simulink model "power_KundurTwoAreaSystem__RTLAB"  (R2021b)
settings: Solver=ode4  StartTime=0.0  StopTime=15  FixedStep=Ts  MaxStep=1/60  RelTol=1e-4
PostLoadFcn:
  | Ts=50e-6; PSSMODEL=1
InitFcn:
  | Ts=50e-6; PSSMODEL=1
undefined symbols (not defined in the file): D1, Delta
libraries: spsGenericPowerSystemStabilizerLib x8, spsThreePhaseVIMeasurementLib x6, spsLoadFlowBusLib x6, spsThreePhaseParallelRLCLoadLib x4, spsThreePhasePISectionLineLib x4, spsSynchronousMachinepuStandardLib x4, spsExcitationSystemLib x4, spsSteamTurbineandGovernorLib x4, spsThreePhaseSeriesRLCLoadLib x4, spsThreePhaseTransformerTwoWindingsLib x4, spsThreePhaseBreakerLib x2, op_dpl_lib x2
(part 1 of 2)
settings Model: ARTEMISmethode_block_infos=$$__separator__$$power_KundurTwoAreaSystem/ARTEMIS Guide$$__separator__$$  Creator=The MathWorks, Inc.  LastModifiedBy=Real_LAB
settings SolverCC: AlgebraicLoopSolver=TrustRegion
settings DataIOCC: SaveOutput=off  SignalLogging=off  DSMLogging=off  SaveTime=off  ReturnWorkspaceOutputs=off  TimeSaveName=t  SignalLoggingName=sigsOut
settings OptimizationCC: BlockReduction=off  BooleanDataType=off  OptimizeBlockIOStorage=off  BufferReuse=off  GlobalBufferReuse=off  ExpressionFolding=off  ExpressionDepthLimit=2147483647  LocalBlockOutputs=off  InitFltsAndDblsToZero=on  LifeSpan=inf  OptimizeDataStoreBuffers=off  BusAssignmentInplaceUpdate=off
settings DebuggingCC: SaveWithParameterizedLinksMsg=none  SignalResolutionControl=TryResolveAllWithWarning  MultiTaskDSMMsg=warning  MultiTaskCondExecSysMsg=none  FcnCallInpInsideContextMsg=warning  UnconnectedOutputMsg=none  StateNameClashWarn=warning  SFUnexpectedBacktrackingDiag=warning  SFNoUnconditionalDefaultTransitionDiag=warning  SFExecutionAtInitializationDiag=none  SFMachineParentedDataDiag=warning  ArithmeticOperatorsInVariantConditions=warning
settings HardwareCC: ProdBitPerPointer=32  ProdBitPerSizeT=32  ProdBitPerPtrDiffT=32  ProdLargestAtomicFloat=None  ProdIntDivRoundTo=Undefined  ProdEndianess=Unspecified  ProdWordSize=32  ProdHWDeviceType=32-bit Generic  TargetBitPerPointer=64  TargetBitPerSizeT=64  TargetBitPerPtrDiffT=64  TargetLongLongMode=on  TargetIntDivRoundTo=Zero  TargetEndianess=LittleEndian  TargetWordSize=64  TargetHWDeviceType=MATLAB Host  ProdEqTarget=off
settings ModelReferenceCC: PropagateSignalLabelsOutOfModel=off
settings SFSimCC: SimUseLocalCustomCode=off  CustomCodeUndefinedFunction=UseInterfaceOnly
settings RTWCC: RTWUseLocalCustomCode=off
settings CodeAppCC: StateflowObjectComments=on
settings GRTTargetCC: TargetFcnLib=ansi_tfl_tmw.mat  TargetLangStandard=C89/C90 (ANSI)  CombineOutputUpdateFcns=off  GRTInterface=on
settings ConfigComp: CovMetricSettings=dw  CovSaveCumulativeToWorkspaceVar=on  CovSaveSingleToWorkspaceVar=on  CovExternalEMLEnable=off  CovSFcnEnable=off
settings SimscapeCC: SimscapeNormalizeSystem=off  SimscapeNominalValues={1, 'bar'; 1, 'cm^3/s'; 1, 'bar*kg/s'; 1, 'kJ/kg'; 1, 'kW'; }

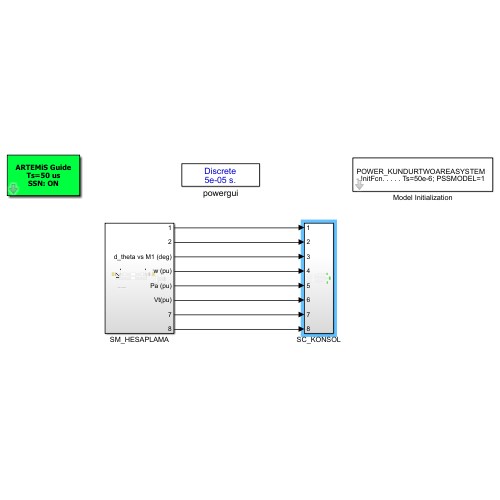
[thumbnail: Simulink's stored preview of the top-level diagram]
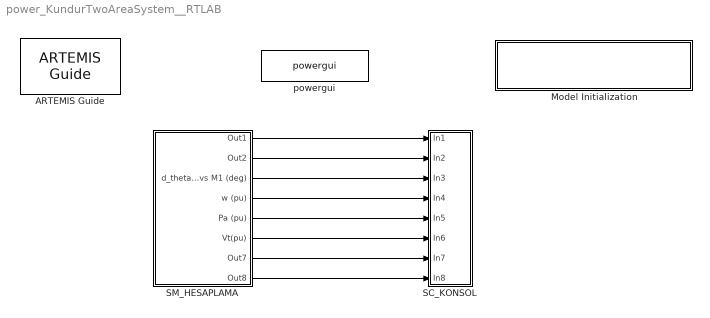
== system power_KundurTwoAreaSystem__RTLAB ==
  ARTEMIS Guide : artemis/ARTEMIS/ARTEMIS Guide  Tag=art7.5  Description=New ARTEMiS block v 7.5b (R2015b+)  lock=on  Ts=Ts  ssn=on  opt=art5  dyna=off  nb_perm=4  RT_fullcomp=off  ssn_itvc=off  ssn_ivic=off  ssn_ext=off  ssn_solver=Art5  iter_type=iSWITCH and iMOV only (default)  ssn_ImpulseLoopBlockedStateUpdate=5  ssn_mov_iter_number=5  ssn_switch_iter_number=3  ssn_lu_or_ldlt=LU (more robust)  ssn_nib_type_verify=on  ssn_use_lu=on  ssn_use_ldlt=off  ssn_impulse=on  ssn_quasimpulse=off  ssn_impulse_loop=5  paraExtinctionThy=off  Thy_Impulse=on  dtc=Off  dtc_opt=normal  ao=off  simtype=off  ct_mac=off  lin_mov=off  lsp=[0.001 2]  spike_skip=Disabled  dtc_extra=1  dtc_sws=normal  dtc_pied=0.5  SPSRulesBlock=SPSRules  tre=off  ctmm=off  LF=off  dpl_type=ARTEMiS DPL  rlc_type=off  custom_type=off  para=on  ssn_full_iteration=off  ssn_init_cond=block only
  Model Initialization : Subsystem  AncestorBlock=artemis/Tools /Misc/Model Initialization  mask(Model Functions){InitFcnX=Ts=50e-6; PSSMODEL=1, prel=off, posl=on, inif=on, strf=off}
      mask prompts: InitFcnX "Initialisation"; prel "Preload Function"; posl "PostLoad Function"; inif "InitFcn"; strf "StartFcn"
      mask init:
      | currentBlock = gcb;
      | root = bdroot(currentBlock);
      | 
      | if ~strcmp(get_param(root,'BlockDiagramType'),'library')
      |     if prel==1
      |         set_param(root, 'PreLoadFcn', InitFcnX);
      |     else
      |         set_param(root, 'PreLoadFcn', '');
      |     end
      |     if inif==1
      |         set_param(root, 'InitFcn', InitFcnX);
      |     else
      |         set_param(root, 'InitFcn', '');
      |     end
      |     if strf==1
      |         set_param(root, 'StartFcn', InitFcnX);
      |     else
      |         set_param(root, 'StartFcn', '');
      |     end
      |     if posl==1
      |         set_param(root, 'PostLoadFcn', InitFcnX);
      |     else
      |         set_param(root, 'PostLoadFcn', '');
      |     end
      | end
      | 
      | pos = get_param(currentBlock, 'Position');
      | width = pos(3) - pos(1); height = pos(4) - pos(2);
      | txt = [ upper(root) '\n' '- InitFcn. . . . . '  get_param(root, 'InitFcn') ];
      settings: CopyFcn=set_param(gcb,'LinkStatus','inactive')
      mask Display: text(5, height*0.5, txt, 'horizontalAlignment', 'left', 'verticalAlignment', 'middle') ;
  SC_KONSOL : Subsystem
  SM_HESAPLAMA : Subsystem
  powergui : spspowerguiLib/powergui  Priority=2  SimulationMode=Discrete  SampleTime=Ts  frequency=60  Iterations=50  frequencyindice=60  Pbase=100e6  ErrMax=1e-4  UnitsV=kV  UnitsW=MW  buscounter=0  FunctionMessages=off  echomessages=off  EnableUseOfTLC=off  CurrentSourceSwitches=off  DisableSnubberDevices=off  DisableRonSwitches=off  DisableVfSwitches=off  DisplayEquations=off  AutomaticDiscreteSolvers=off  SolverType=Tustin  Interpol=off  ExternalGateDelay=off  methode=off  Ts=0  x0status=blocks  SPID=off  SwTol=0  HookPort=off  NonlinearTolerance=1e-4  nMaxIteration=100  ContinueOnMaxIteration=off  RestoreLinks=warning  ResistiveCurrentMeasurement=off  Frange=logspace(0,3,50)  Ylog=off  Xlog=off  ShowGrid=off  save=off  variable=ZData  structure=0  ZoomFFT=on  StartTime=0.0  cycles=1  DisplayStyle=1  fundamental=60  FreqAxis=off  MaxFrequency=1000  frequencyindicesteady=1  RmsSteady=1  display=off
  wires:
  SM_HESAPLAMA/1(Out1) -> SC_KONSOL/1(In1)
  SM_HESAPLAMA/2(Out2) -> SC_KONSOL/2(In2)
  SM_HESAPLAMA/3(d_theta vs M1 (deg)) -> SC_KONSOL/3(In3)
  SM_HESAPLAMA/4(w (pu)) -> SC_KONSOL/4(In4)
  SM_HESAPLAMA/5(Pa (pu)) -> SC_KONSOL/5(In5)
  SM_HESAPLAMA/6(Vt(pu)) -> SC_KONSOL/6(In6)
  SM_HESAPLAMA/7(Out7) -> SC_KONSOL/7(In7)
  SM_HESAPLAMA/8(Out8) -> SC_KONSOL/8(In8)

== system power_KundurTwoAreaSystem__RTLAB/Model Initialization ==

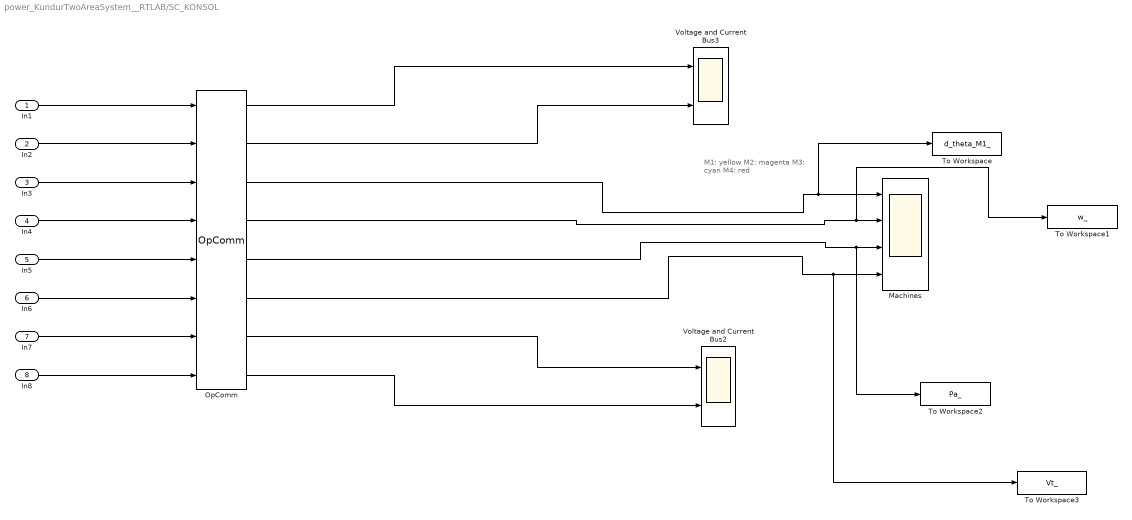
== system power_KundurTwoAreaSystem__RTLAB/SC_KONSOL ==
  note: M1: yellow
      | M2: magenta
      | M3: cyan
      | M4: red
  In1 : Inport
  In2 : Inport  Port=2
  In3 : Inport  Port=3
  In4 : Inport  Port=4
  In5 : Inport  Port=5
  In6 : Inport  Port=6
  In7 : Inport  Port=7
  In8 : Inport  Port=8
  Machines : Scope  NumInputPorts=4
  OpComm : rtlab/OpComm  nbport=8  groupe_acq=1  subsys_rate=0  st=0  Synchronization=on  Interpolation=on  Threshold=1.0  Missed_Data=off  Sim_Time=off  Samples=off  dynSigOut=off  from_console=0  warning_done=off  writeOpCommFile=off  Offset=off
      settings: SourceProductName=RT-LAB
  To Workspace : ToWorkspace  VariableName=d_theta_M1_  SaveFormat=Timeseries  SampleTime=-1
  To Workspace1 : ToWorkspace  VariableName=w_  SaveFormat=Timeseries  SampleTime=-1
  To Workspace2 : ToWorkspace  VariableName=Pa_  SaveFormat=Timeseries  SampleTime=-1
  To Workspace3 : ToWorkspace  VariableName=Vt_  SaveFormat=Timeseries  SampleTime=-1
  Voltage and Current Bus2 : Scope  NumInputPorts=2
  Voltage and Current Bus3 : Scope  NumInputPorts=2
  wires:
  In1/1 -> OpComm/1
  In2/1 -> OpComm/2
  In3/1 -> OpComm/3
  In4/1 -> OpComm/4
  In5/1 -> OpComm/5
  In6/1 -> OpComm/6
  In7/1 -> OpComm/7
  In8/1 -> OpComm/8
  OpComm/8 -> Voltage and Current Bus2/2
  OpComm/7 -> Voltage and Current Bus2/1
  OpComm/1 -> Voltage and Current Bus3/1
  OpComm/2 -> Voltage and Current Bus3/2
  OpComm/3 -> To Workspace/1, Machines/1
  OpComm/4 -> To Workspace1/1, Machines/2
  OpComm/5 -> To Workspace2/1, Machines/3
  OpComm/6 -> To Workspace3/1, Machines/4

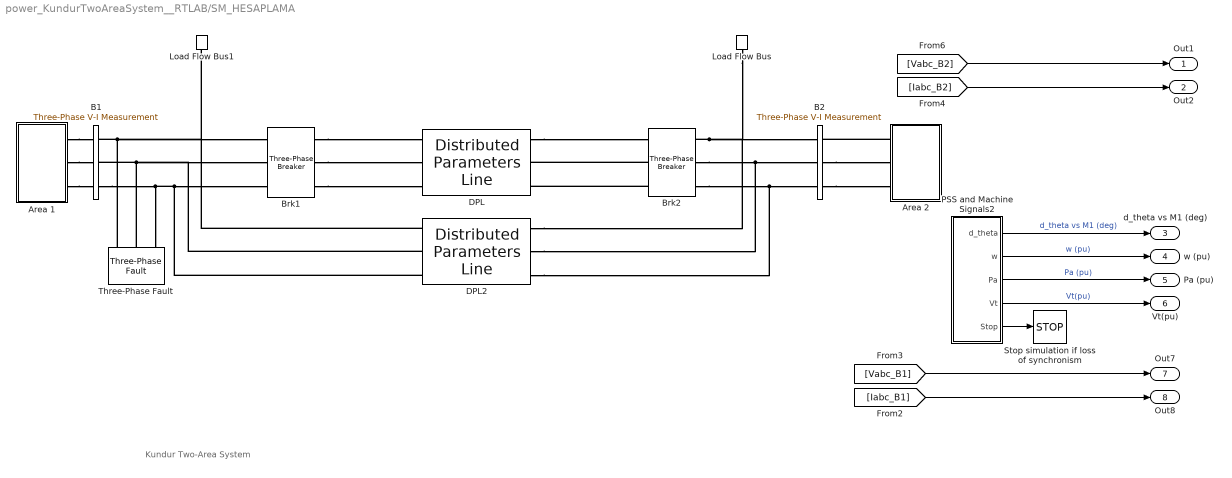
== system power_KundurTwoAreaSystem__RTLAB/SM_HESAPLAMA ==
  note: Kundur Two-Area System
  " Brk2" : spsThreePhaseBreakerLib/Three-Phase Breaker  InitialState=closed  SwitchA=on  SwitchB=on  SwitchC=on  SwitchTimes=[2+12]*100  External=off  BreakerResistance=0.001  SnubberResistance=1e6  SnubberCapacitance=0  Measurements=None
      settings: AttributesFormatString=\n
  Area 1 : Subsystem
  Area 2 : Subsystem
  B1 : spsThreePhaseVIMeasurementLib/Three-Phase V-I Measurement  VoltageMeasurement=phase-to-ground  SetLabelV=on  LabelV=Vabc_B1  Vpu=on  VpuLL=off  CurrentMeasurement=yes  SetLabelI=on  LabelI=Iabc_B1  Ipu=off  Pbase=100e6  Vbase=230e3  OutputType=Complex  PhasorSimulation=off  PSBequivalent=0
  B2 : spsThreePhaseVIMeasurementLib/Three-Phase V-I Measurement  VoltageMeasurement=phase-to-ground  SetLabelV=on  LabelV=Vabc_B2  Vpu=off  VpuLL=off  CurrentMeasurement=yes  SetLabelI=on  LabelI=Iabc_B2  Ipu=off  Pbase=100e6  Vbase=500e3  OutputType=Complex  PhasorSimulation=off  PSBequivalent=0
  Brk1 : spsThreePhaseBreakerLib/Three-Phase Breaker  InitialState=closed  SwitchA=off  SwitchB=off  SwitchC=off  SwitchTimes=[2+12]  External=off  BreakerResistance=0.001  SnubberResistance=inf  SnubberCapacitance=0  Measurements=None
      settings: AttributesFormatString=\n
  DPL : op_dpl_lib/Distributed Parameters Line  SimulationMode=ARTEMIS model  Phases=3  Frequency=60  Resistance=[0.0001*529 1.61]  Inductance=[0.001*529/(377) 0.0061]  Capacitance=[0.00175/529/(377) 5.2489e-9]  Length=220  Measurements=None
  DPL2 : op_dpl_lib/Distributed Parameters Line  SimulationMode=ARTEMIS model  Phases=3  Frequency=60  Resistance=[0.0001*529 1.61]  Inductance=[0.001*529/(377) 0.0061]  Capacitance=[0.00175/529/(377) 5.2489e-9]  Length=220  Measurements=None
  Load Flow Bus : spsLoadFlowBusLib/Load Flow Bus  LConnTagsString=a  Phases=single  Connectors=on one side  ID=B2  Vbase=230e3  Vref=1  Vangle=0  VLF=1.003  VLFb=1  VLFc=1  angleLF=-11.54  angleLFb=0  angleLFc=0
      settings: AttributesFormatString=%<ID>\n%<Vbase>V\n%<VLF>pu\n%<angleLF>deg.  SourceProductBaseCode=PS
  Load Flow Bus1 : spsLoadFlowBusLib/Load Flow Bus  LConnTagsString=a  Phases=single  Connectors=on one side  ID=B1  Vbase=230e3  Vref=1  Vangle=0  VLF=0.9914  VLFb=1  VLFc=1  angleLF=15.04  angleLFb=0  angleLFc=0
      settings: AttributesFormatString=%<ID>\n%<Vbase>V\n%<VLF>pu\n%<angleLF>deg.  SourceProductBaseCode=PS
  PSS and Machine Signals2 : Subsystem
  Stop simulation if loss of synchronism : Stop
  Three-Phase Fault : spsThreePhaseFaultLib/Three-Phase Fault  InitialStates=0  FaultA=on  FaultB=on  FaultC=on  GroundFault=on  SwitchTimes=[2 2.1]  External=off  SwitchStatus=NaN  FaultResistance=0.001  GroundResistance=0.001  SnubberResistance=1e6  SnubberCapacitance=inf  Measurements=None
  Out1 : Outport
  Out2 : Outport  Port=2
  d_theta vs M1 (deg) : Outport  Port=3
  w (pu) : Outport  Port=4
  Pa (pu) : Outport  Port=5
  Vt(pu) : Outport  Port=6
  Out7 : Outport  Port=7
  Out8 : Outport  Port=8
  wires:
  [Vabc_B2] -> Out1/1
  PSS and Machine Signals2/1(d_theta) -> d_theta vs M1 (deg)/1  "d_theta vs M1 (deg)"
  PSS and Machine Signals2/4(Vt) -> Vt(pu)/1  "Vt(pu)"
  PSS and Machine Signals2/2(w) -> w (pu)/1  "w (pu)"
  PSS and Machine Signals2/5(Stop) -> Stop simulation if loss of synchronism/1
  [Iabc_B1] -> Out8/1
  [Vabc_B1] -> Out7/1
  [Iabc_B2] -> Out2/1
  PSS and Machine Signals2/3(Pa) -> Pa (pu)/1  "Pa (pu)"
  connections:
  B2/RConn2 -- Area 2/LConn2
  " Brk2"/LConn2 -- DPL/RConn2
  B2/RConn3 -- Area 2/LConn3
  " Brk2"/RConn1 -- DPL2/RConn1 -- Load Flow Bus/LConn1 -- B2/LConn1
  " Brk2"/RConn2 -- DPL2/RConn2 -- B2/LConn2
  Area 1/RConn3 -- B1/LConn3
  Area 1/RConn1 -- B1/LConn1
  Brk1/RConn3 -- DPL/LConn3
  DPL2/LConn1 -- Brk1/LConn1 -- Load Flow Bus1/LConn1 -- Three-Phase Fault/LConn1 -- B1/RConn1
  Brk1/RConn1 -- DPL/LConn1
  Area 2/LConn1 -- B2/RConn1
  DPL2/LConn3 -- B1/RConn3 -- Three-Phase Fault/LConn3 -- Brk1/LConn3
  " Brk2"/LConn3 -- DPL/RConn3
  " Brk2"/RConn3 -- DPL2/RConn3 -- B2/LConn3
  DPL/RConn1 -- " Brk2"/LConn1
  DPL2/LConn2 -- Brk1/LConn2 -- Three-Phase Fault/LConn2 -- B1/RConn2
  Brk1/RConn2 -- DPL/LConn2
  Area 1/RConn2 -- B1/LConn2

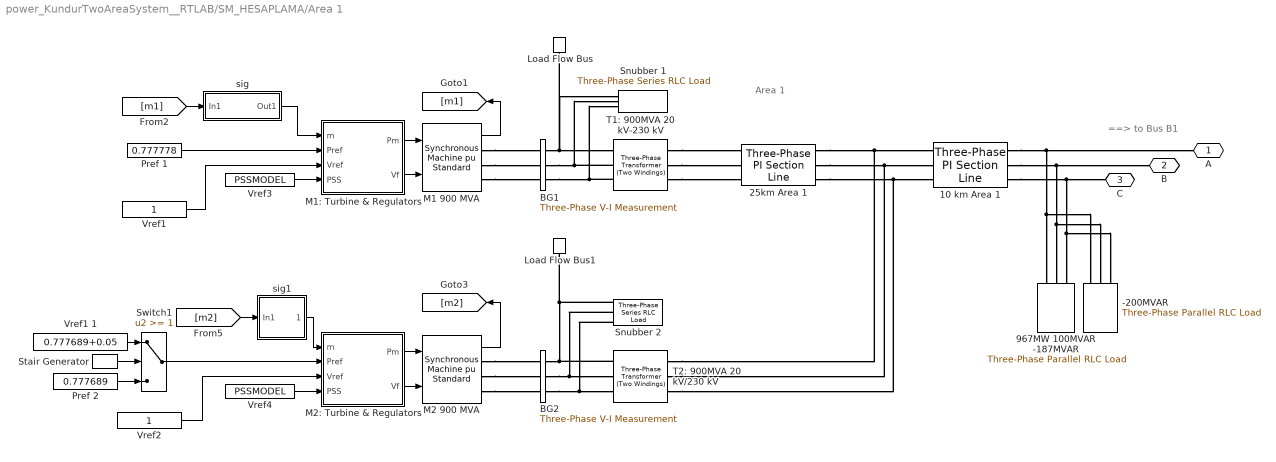
== system power_KundurTwoAreaSystem__RTLAB/SM_HESAPLAMA/Area 1 ==
  note: Area 1
  note: ==> to Bus B1
  -200MVAR : spsThreePhaseParallelRLCLoadLib/Three-Phase Parallel RLC Load  LConnTagsString=A|B|C  Configuration=Y (grounded)  NominalVoltage=230e3  Vabc=[1e3 1e3 1e3]  Vabcp=[1e3 1e3 1e3]  NominalFrequency=60  UnbalancedPower=off  ActivePower=0  InductivePower=0  CapacitivePower=200e6  Pabc=[10e3 9e3 11e3]  QLabc=[100 90 110]  QCabc=[100 90 110]  Pabcp=[10e3 9e3 11e3]  QLabcp=[100 90 110]  QCabcp=[100 90 110]  Measurements=None  LoadType=constant Z
  10 km Area 1 : spsThreePhasePISectionLineLib/Three-Phase PI Section Line  LConnTagsString=a|b|c  RConnTagsString=A|B|C  Length=10  Frequency=60  Resistances=[0.0001*529 1.61]  Inductances=[0.001*529/(377) 0.0061]  Capacitances=[0.00175/529/(377) 5.2489e-9]
  25km Area 1 : spsThreePhasePISectionLineLib/Three-Phase PI Section Line  LConnTagsString=a|b|c  RConnTagsString=A|B|C  Length=25  Frequency=60  Resistances=[0.0001*529 1.61]  Inductances=[0.001*529/(377) 0.0061]  Capacitances=[0.00175/529/(377) 5.2489e-9]
  967MW 100MVAR -187MVAR : spsThreePhaseParallelRLCLoadLib/Three-Phase Parallel RLC Load  LConnTagsString=A|B|C  Configuration=Y (grounded)  NominalVoltage=230e3  Vabc=[1e3 1e3 1e3]  Vabcp=[1e3 1e3 1e3]  NominalFrequency=60  UnbalancedPower=off  ActivePower=967e6  InductivePower=100e6  CapacitivePower=187e6  Pabc=[10e3 9e3 11e3]  QLabc=[100 90 110]  QCabc=[100 90 110]  Pabcp=[10e3 9e3 11e3]  QLabcp=[100 90 110]  QCabcp=[100 90 110]  Measurements=None  LoadType=constant Z
  BG1 : spsThreePhaseVIMeasurementLib/Three-Phase V-I Measurement  VoltageMeasurement=phase-to-ground  SetLabelV=on  LabelV=Vabc_G1  Vpu=on  VpuLL=off  CurrentMeasurement=yes  SetLabelI=on  LabelI=Iabc_G1  Ipu=on  Pbase=900e6  Vbase=20e3  OutputType=Complex  PhasorSimulation=off  PSBequivalent=0
  BG2 : spsThreePhaseVIMeasurementLib/Three-Phase V-I Measurement  VoltageMeasurement=no  SetLabelV=on  LabelV=Vabc_G2  Vpu=on  VpuLL=off  CurrentMeasurement=no  SetLabelI=on  LabelI=Iabc_G2  Ipu=on  Pbase=900e6  Vbase=20e3  OutputType=Complex  PhasorSimulation=off  PSBequivalent=0
  Load Flow Bus : spsLoadFlowBusLib/Load Flow Bus  LConnTagsString=a  Phases=single  Connectors=on one side  ID=M1_Area1  Vbase=20e3  Vref=1  Vangle=0  VLF=1  VLFb=1  VLFc=1  angleLF=10.19  angleLFb=0  angleLFc=0
      settings: AttributesFormatString=%<ID>\n%<Vbase>V\n%<VLF>pu\n%<angleLF>deg.  SourceProductBaseCode=PS
  Load Flow Bus1 : spsLoadFlowBusLib/Load Flow Bus  LConnTagsString=a  Phases=single  Connectors=on one side  ID=M2_Area1  Vbase=20e3  Vref=1  Vangle=0  VLF=1  VLFb=1  VLFc=1  angleLF=0  angleLFb=0  angleLFc=0
      settings: AttributesFormatString=%<ID>\n%<Vbase>V\n%<VLF>pu\n%<angleLF>deg.  SourceProductBaseCode=PS
  M1 900 MVA : spsSynchronousMachinepuStandardLib/Synchronous Machine pu Standard  PresetModel=No  MechanicalLoad=Mechanical power Pm  ShowDetailedParameters=on  RotorType=Round  Units=per unit standard parameters  MeasurementBus=off  NominalParameters="[900E6  20000   60 ]"  Reactances1=[1.8 .3 .25 1.7 .55 .25 .2]  Reactances2=[ 1.305, 0.296, 0.252, 0.474, 0.243, 0.18 ]  dAxisTimeConstants=Open-circuit  qAxisTimeConstants=Open-circuit  TimeConstants1=[]  TimeConstants2=[8 .03 .4 .05]  TimeConstants3=[]  TimeConstants4=[]  TimeConstants5=[ 1.01, 0.053, 0.1 ]  TimeConstants6=[]  TimeConstants7=[]  TimeConstants8=[]  StatorResistance=0.0025  Mechanical="[ 6.5 0  4]"  PolePairs=4  InitialConditions=[0 -31.4247 0.784453 0.784453 0.784453 2.7401 -117.26 122.74 1.83395]  SetSaturation=off  Saturation=[0.6404,0.7127,0.8441,0.9214,0.9956,1.082,1.19,1.316,1.457;0.7,0.7698,0.8872,0.9466,0.9969,1.046,1.1,1.151,1.201]  LoadFlowParameters=[1 700000000 0 0 0]  TsPowergui=0  TsBlock=-1  IterativeModel=Trapezoidal non iterative  IterativeDiscreteModel=Trapezoidal non iterative  BusType=PV  Pref=700000000  Qref=0  Qmin=-inf  Qmax=inf  PLF=0  QLF=0
      settings: SourceProductBaseCode=PS
  M1: Turbine & Regulators : Subsystem
  M2 900 MVA : spsSynchronousMachinepuStandardLib/Synchronous Machine pu Standard  PresetModel=No  MechanicalLoad=Mechanical power Pm  ShowDetailedParameters=on  RotorType=Round  Units=per unit standard parameters  MeasurementBus=off  NominalParameters="[900E6  20000   60 ]"  Reactances1=[1.8 .3 .25 1.7 .55 .25 .2]  Reactances2=[ 1.305, 0.296, 0.252, 0.474, 0.243, 0.18 ]  dAxisTimeConstants=Open-circuit  qAxisTimeConstants=Open-circuit  TimeConstants1=[]  TimeConstants2=[8 .03 .4 .05]  TimeConstants3=[]  TimeConstants4=[]  TimeConstants5=[ 1.01, 0.053, 0.1 ]  TimeConstants6=[]  TimeConstants7=[]  TimeConstants8=[]  StatorResistance=0.0025  Mechanical="[ 6.5 0  4]"  PolePairs=4  InitialConditions=[0 -42.8075 0.788608 0.788608 0.788608 -9.54571 -129.546 110.454 1.86756]  SetSaturation=off  Saturation=[0.6404,0.7127,0.8441,0.9214,0.9956,1.082,1.19,1.316,1.457;0.7,0.7698,0.8872,0.9466,0.9969,1.046,1.1,1.151,1.201]  LoadFlowParameters=[2 700000000 0 0 0]  TsPowergui=0  TsBlock=-1  IterativeModel=Trapezoidal non iterative  IterativeDiscreteModel=Trapezoidal non iterative  BusType=swing  Pref=0  Qref=0  Qmin=-inf  Qmax=inf  PLF=0  QLF=0
      settings: SourceProductBaseCode=PS
  M2: Turbine & Regulators : Subsystem
  Pref 1 : Constant  Value=0.777778
  Pref 2 : Constant  Value=0.777689
  Snubber 1 : spsThreePhaseSeriesRLCLoadLib/Three-Phase Series RLC Load  LConnTagsString=A|B|C  Configuration=Y (grounded)  NominalVoltage=20000  Vabc=[1e3 1e3 1e3]  Vabcp=[1e3 1e3 1e3]  NominalFrequency=60  UnbalancedPower=off  ActivePower=1e6  InductivePower=0  CapacitivePower=1e7  Pabc=[10e3 9e3 11e3]  QLabc=[100 90 110]  QCabc=[100 90 110]  Pabcp=[10e3 9e3 11e3]  QLabcp=[100 90 110]  QCabcp=[100 90 110]  Measurements=None  LoadType=constant Z
  Snubber 2 : spsThreePhaseSeriesRLCLoadLib/Three-Phase Series RLC Load  LConnTagsString=A|B|C  Configuration=Y (grounded)  NominalVoltage=20000  Vabc=[1e3 1e3 1e3]  Vabcp=[1e3 1e3 1e3]  NominalFrequency=60  UnbalancedPower=off  ActivePower=1e6  InductivePower=0  CapacitivePower=1e7  Pabc=[10e3 9e3 11e3]  QLabc=[100 90 110]  QCabc=[100 90 110]  Pabcp=[10e3 9e3 11e3]  QLabcp=[100 90 110]  QCabcp=[100 90 110]  Measurements=None  LoadType=constant Z
  Stair Generator : spsStairGeneratorLib/Stair Generator  t=[0 15 20]  e=[0 1 0 ]  Ts=0
  Switch1 : Switch  Threshold=1  InputSameDT=on
  T1: 900MVA 20 kV-230 kV : spsThreePhaseTransformerTwoWindingsLib/Three-Phase Transformer (Two Windings)  Winding1Connection=Delta (D1)  Winding2Connection=Yg  CoreType=Three single-phase transformers  SetSaturation=off  Hysteresis=off  DataFile='hysteresis'  SetInitialFlux=off  Measurements=None  UNITS=pu  NominalPower="[ 900e6   60 ]"  Winding1="[ 20e3  1e-6   0  ]"  Winding2="[ 230e3  1e-6   0.15 ]"  Rm=500  Lm=500  L0=0.5  Saturation="[ 0,0  ;  0.005,1.2  ;  1.0,1.4 ]"  InitialFluxes=[ 0.8 , -0.8 , 0.7 ]  BreakLoop=off  DiscreteSolver=Trapezoidal iterative  DataType=off  TransfoNumber=0
  T2: 900MVA 20 kV/230 kV : spsThreePhaseTransformerTwoWindingsLib/Three-Phase Transformer (Two Windings)  Winding1Connection=Delta (D1)  Winding2Connection=Yg  CoreType=Three single-phase transformers  SetSaturation=off  Hysteresis=off  DataFile='hysteresis'  SetInitialFlux=off  Measurements=None  UNITS=pu  NominalPower=[ 900e6 60 ]  Winding1="[ 20e3 1e-6  0.0]"  Winding2=[ 230e3 1e-6 0.15]  Rm=500  Lm=500  L0=0.5  Saturation="[ 0,0  ;  0.005,1.2  ;  1.0,1.4 ]"  InitialFluxes=[ 0.8 , -0.8 , 0.7 ]  BreakLoop=off  DiscreteSolver=Trapezoidal iterative  DataType=off  TransfoNumber=0
  Vref1 : Constant
  Vref1 1 : Constant  Value=0.777689+0.05
  Vref2 : Constant
  Vref3 : Constant  Value=PSSMODEL
  Vref4 : Constant  Value=PSSMODEL
  sig : Subsystem
  sig1 : Subsystem
  " A" : PMIOPort  Side=Right
  " B" : PMIOPort  Port=2  Side=Right
  " C" : PMIOPort  Port=3  Side=Right
  wires:
  Pref 1/1 -> M1: Turbine & Regulators/2(Pref)
  Vref2/1 -> M2: Turbine & Regulators/3(Vref)
  Vref4/1 -> M2: Turbine & Regulators/4(PSS)
  sig/1(Out1) -> M1: Turbine & Regulators/1(m)
  M1 900 MVA/1 -> [m1]
  M2 900 MVA/1 -> [m2]
  [m1] -> sig/1(In1)
  Vref3/1 -> M1: Turbine & Regulators/4(PSS)
  sig1/1(Out1) -> M2: Turbine & Regulators/1(m)
  [m2] -> sig1/1(In1)
  Stair Generator/1 -> Switch1/2
  Pref 2/1 -> Switch1/3
  Vref1 1/1 -> Switch1/1
  Switch1/1 -> M2: Turbine & Regulators/2(Pref)
  Vref1/1 -> M1: Turbine & Regulators/3(Vref)
  M1: Turbine & Regulators/1(Pm) -> M1 900 MVA/1
  M1: Turbine & Regulators/2(Vf) -> M1 900 MVA/2
  M2: Turbine & Regulators/2(Vf) -> M2 900 MVA/2
  M2: Turbine & Regulators/1(Pm) -> M2 900 MVA/1
  connections:
  T1: 900MVA 20 kV-230 kV/RConn1 -- 25km Area 1/LConn1
  T1: 900MVA 20 kV-230 kV/RConn2 -- 25km Area 1/LConn2
  Snubber 2/LConn1 -- T2: 900MVA 20 kV/230 kV/LConn1 -- BG2/RConn1 -- Load Flow Bus1/LConn1
  Snubber 2/LConn2 -- T2: 900MVA 20 kV/230 kV/LConn2 -- BG2/RConn2
  Snubber 2/LConn3 -- BG2/RConn3 -- T2: 900MVA 20 kV/230 kV/LConn3
  T1: 900MVA 20 kV-230 kV/RConn3 -- 25km Area 1/LConn3
  10 km Area 1/RConn1 -- " A"/RConn1 -- 967MW 100MVAR -187MVAR/LConn1 -- -200MVAR/LConn1
  10 km Area 1/RConn2 -- " B"/RConn1 -- 967MW 100MVAR -187MVAR/LConn2 -- -200MVAR/LConn2
  10 km Area 1/RConn3 -- " C"/RConn1 -- 967MW 100MVAR -187MVAR/LConn3 -- -200MVAR/LConn3
  Snubber 1/LConn1 -- Load Flow Bus/LConn1 -- T1: 900MVA 20 kV-230 kV/LConn1 -- BG1/RConn1
  T1: 900MVA 20 kV-230 kV/LConn2 -- Snubber 1/LConn2 -- BG1/RConn2
  T1: 900MVA 20 kV-230 kV/LConn3 -- Snubber 1/LConn3 -- BG1/RConn3
  25km Area 1/RConn2 -- 10 km Area 1/LConn2 -- T2: 900MVA 20 kV/230 kV/RConn2
  25km Area 1/RConn1 -- 10 km Area 1/LConn1 -- T2: 900MVA 20 kV/230 kV/RConn1
  25km Area 1/RConn3 -- 10 km Area 1/LConn3 -- T2: 900MVA 20 kV/230 kV/RConn3
  M1 900 MVA/RConn1 -- BG1/LConn1
  M1 900 MVA/RConn2 -- BG1/LConn2
  M1 900 MVA/RConn3 -- BG1/LConn3
  M2 900 MVA/RConn1 -- BG2/LConn1
  M2 900 MVA/RConn2 -- BG2/LConn2
  M2 900 MVA/RConn3 -- BG2/LConn3

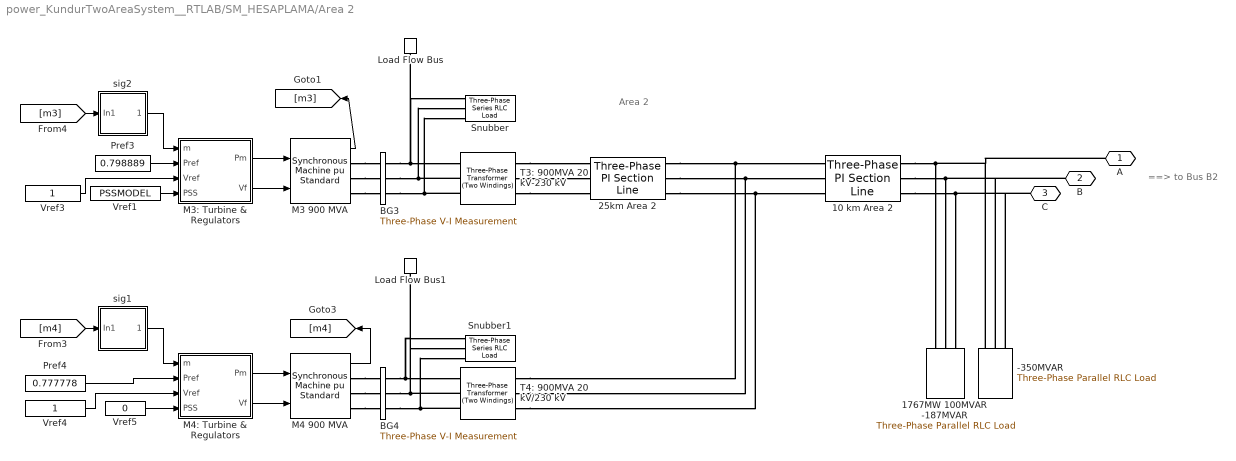
== system power_KundurTwoAreaSystem__RTLAB/SM_HESAPLAMA/Area 2 ==
  note: ==> to Bus B2
  note: Area 2
  -350MVAR : spsThreePhaseParallelRLCLoadLib/Three-Phase Parallel RLC Load  LConnTagsString=A|B|C  Configuration=Y (grounded)  NominalVoltage=230e3  Vabc=[1e3 1e3 1e3]  Vabcp=[1e3 1e3 1e3]  NominalFrequency=60  UnbalancedPower=off  ActivePower=0  InductivePower=0  CapacitivePower=350e6  Pabc=[10e3 9e3 11e3]  QLabc=[100 90 110]  QCabc=[100 90 110]  Pabcp=[10e3 9e3 11e3]  QLabcp=[100 90 110]  QCabcp=[100 90 110]  Measurements=None  LoadType=constant Z
  10 km Area 2 : spsThreePhasePISectionLineLib/Three-Phase PI Section Line  LConnTagsString=a|b|c  RConnTagsString=A|B|C  Length=10  Frequency=60  Resistances=[0.0001*529 1.61]  Inductances=[0.001*529/(377) 0.0061]  Capacitances=[0.00175/529/(377) 5.2489e-9]
  1767MW 100MVAR -187MVAR : spsThreePhaseParallelRLCLoadLib/Three-Phase Parallel RLC Load  LConnTagsString=A|B|C  Configuration=Y (grounded)  NominalVoltage=230e3  Vabc=[1e3 1e3 1e3]  Vabcp=[1e3 1e3 1e3]  NominalFrequency=60  UnbalancedPower=off  ActivePower=1767e6  InductivePower=100e6  CapacitivePower=187e6  Pabc=[10e3 9e3 11e3]  QLabc=[100 90 110]  QCabc=[100 90 110]  Pabcp=[10e3 9e3 11e3]  QLabcp=[100 90 110]  QCabcp=[100 90 110]  Measurements=None  LoadType=constant Z
  25km Area 2 : spsThreePhasePISectionLineLib/Three-Phase PI Section Line  LConnTagsString=a|b|c  RConnTagsString=A|B|C  Length=25  Frequency=60  Resistances=[0.0001*529 1.61]  Inductances=[0.001*529/(377) 0.0061]  Capacitances=[0.00175/529/(377) 5.2489e-9]
  BG3 : spsThreePhaseVIMeasurementLib/Three-Phase V-I Measurement  VoltageMeasurement=no  SetLabelV=on  LabelV=Vabc_G3  Vpu=on  VpuLL=off  CurrentMeasurement=no  SetLabelI=on  LabelI=Iabc_G3  Ipu=on  Pbase=900e6  Vbase=20e3  OutputType=Complex  PhasorSimulation=off  PSBequivalent=0
  BG4 : spsThreePhaseVIMeasurementLib/Three-Phase V-I Measurement  VoltageMeasurement=no  SetLabelV=on  LabelV=Vabc_G4  Vpu=on  VpuLL=off  CurrentMeasurement=no  SetLabelI=on  LabelI=Iabc_G4  Ipu=on  Pbase=900e6  Vbase=20e3  OutputType=Complex  PhasorSimulation=off  PSBequivalent=0
  Load Flow Bus : spsLoadFlowBusLib/Load Flow Bus  LConnTagsString=a  Phases=single  Connectors=on one side  ID=M3_Area2  Vbase=20e3  Vref=1  Vangle=0  VLF=1  VLFb=1  VLFc=1  angleLF=-16.02  angleLFb=0  angleLFc=0
      settings: AttributesFormatString=%<ID>\n%<Vbase>V\n%<VLF>pu\n%<angleLF>deg.  SourceProductBaseCode=PS
  Load Flow Bus1 : spsLoadFlowBusLib/Load Flow Bus  LConnTagsString=a  Phases=single  Connectors=on one side  ID=M4_Area2  Vbase=20e3  Vref=1  Vangle=0  VLF=1  VLFb=1  VLFc=1  angleLF=-26.66  angleLFb=0  angleLFc=0
      settings: AttributesFormatString=%<ID>\n%<Vbase>V\n%<VLF>pu\n%<angleLF>deg.  SourceProductBaseCode=PS
  M3 900 MVA : spsSynchronousMachinepuStandardLib/Synchronous Machine pu Standard  PresetModel=No  MechanicalLoad=Mechanical power Pm  ShowDetailedParameters=on  RotorType=Round  Units=per unit standard parameters  MeasurementBus=off  NominalParameters="[900E6  20000   60 ]"  Reactances1=[1.8 .3 .25 1.7 .55 .25 .2]  Reactances2=[ 1.305, 0.296, 0.252, 0.474, 0.243, 0.18 ]  dAxisTimeConstants=Open-circuit  qAxisTimeConstants=Open-circuit  TimeConstants1=[]  TimeConstants2=[8 .03 .4 .05]  TimeConstants3=[]  TimeConstants4=[]  TimeConstants5=[ 1.01, 0.053, 0.1 ]  TimeConstants6=[]  TimeConstants7=[]  TimeConstants8=[]  StatorResistance=0.0025  Mechanical="[ 6.175 0  4]"  PolePairs=4  InitialConditions=[0 -56.3243 0.8041 0.8041 0.8041 -22.4087 -142.409 97.5913 1.85092]  SetSaturation=off  Saturation=[0.6404,0.7127,0.8441,0.9214,0.9956,1.082,1.19,1.316,1.457;0.7,0.7698,0.8872,0.9466,0.9969,1.046,1.1,1.151,1.201]  LoadFlowParameters=[1 719000000 0 0 0]  TsPowergui=0  TsBlock=-1  IterativeModel=Trapezoidal non iterative  IterativeDiscreteModel=Trapezoidal non iterative  BusType=PV  Pref=719000000  Qref=0  Qmin=-inf  Qmax=inf  PLF=0  QLF=0
      settings: SourceProductBaseCode=PS
  M3: Turbine & Regulators : Subsystem
  M4 900 MVA : spsSynchronousMachinepuStandardLib/Synchronous Machine pu Standard  PresetModel=No  MechanicalLoad=Mechanical power Pm  ShowDetailedParameters=on  RotorType=Round  Units=per unit standard parameters  MeasurementBus=off  NominalParameters="[900E6  20000   60 ]"  Reactances1=[1.8 .3 .25 1.7 .55 .25 .2]  Reactances2=[ 1.305, 0.296, 0.252, 0.474, 0.243, 0.18 ]  dAxisTimeConstants=Open-circuit  qAxisTimeConstants=Open-circuit  TimeConstants1=[]  TimeConstants2=[8 .03 .4 .05]  TimeConstants3=[]  TimeConstants4=[]  TimeConstants5=[ 1.01, 0.053, 0.1 ]  TimeConstants6=[]  TimeConstants7=[]  TimeConstants8=[]  StatorResistance=0.0025  Mechanical="[ 6.175 0  4]"  PolePairs=4  InitialConditions=[0 -67.7513 0.783185 0.783185 0.783185 -33.268 -153.268 86.732 1.82209]  SetSaturation=off  Saturation=[0.6404,0.7127,0.8441,0.9214,0.9956,1.082,1.19,1.316,1.457;0.7,0.7698,0.8872,0.9466,0.9969,1.046,1.1,1.151,1.201]  LoadFlowParameters=[1 700000000 0 0 0]  TsPowergui=0  TsBlock=-1  IterativeModel=Trapezoidal non iterative  IterativeDiscreteModel=Trapezoidal non iterative  BusType=PV  Pref=700000000  Qref=0  Qmin=-inf  Qmax=inf  PLF=0  QLF=0
      settings: SourceProductBaseCode=PS
  M4: Turbine & Regulators : Subsystem
  Pref3 : Constant  Value=0.798889
  Pref4 : Constant  Value=0.777778
  Snubber : spsThreePhaseSeriesRLCLoadLib/Three-Phase Series RLC Load  LConnTagsString=A|B|C  Configuration=Y (grounded)  NominalVoltage=20000  Vabc=[1e3 1e3 1e3]  Vabcp=[1e3 1e3 1e3]  NominalFrequency=60  UnbalancedPower=off  ActivePower=1e6  InductivePower=0  CapacitivePower=1e7  Pabc=[10e3 9e3 11e3]  QLabc=[100 90 110]  QCabc=[100 90 110]  Pabcp=[10e3 9e3 11e3]  QLabcp=[100 90 110]  QCabcp=[100 90 110]  Measurements=None  LoadType=constant Z
  Snubber1 : spsThreePhaseSeriesRLCLoadLib/Three-Phase Series RLC Load  LConnTagsString=A|B|C  Configuration=Y (grounded)  NominalVoltage=20000  Vabc=[1e3 1e3 1e3]  Vabcp=[1e3 1e3 1e3]  NominalFrequency=60  UnbalancedPower=off  ActivePower=1e6  InductivePower=0  CapacitivePower=1e7  Pabc=[10e3 9e3 11e3]  QLabc=[100 90 110]  QCabc=[100 90 110]  Pabcp=[10e3 9e3 11e3]  QLabcp=[100 90 110]  QCabcp=[100 90 110]  Measurements=None  LoadType=constant Z
  T3: 900MVA 20 kV-230 kV : spsThreePhaseTransformerTwoWindingsLib/Three-Phase Transformer (Two Windings)  Winding1Connection=Delta (D1)  Winding2Connection=Yg  CoreType=Three single-phase transformers  SetSaturation=off  Hysteresis=off  DataFile='hysteresis'  SetInitialFlux=off  Measurements=None  UNITS=pu  NominalPower="[ 900e6   60 ]"  Winding1="[ 20e3  1e-6   0  ]"  Winding2="[ 230e3  1e-6   0.15 ]"  Rm=500  Lm=500  L0=0.5  Saturation="[ 0,0  ;  0.005,1.2  ;  1.0,1.4 ]"  InitialFluxes=[ 0.8 , -0.8 , 0.7 ]  BreakLoop=off  DiscreteSolver=Trapezoidal iterative  DataType=off  TransfoNumber=0
  T4: 900MVA 20 kV/230 kV : spsThreePhaseTransformerTwoWindingsLib/Three-Phase Transformer (Two Windings)  Winding1Connection=Delta (D1)  Winding2Connection=Yg  CoreType=Three single-phase transformers  SetSaturation=off  Hysteresis=off  DataFile='hysteresis'  SetInitialFlux=off  Measurements=None  UNITS=pu  NominalPower=[ 900e6 60 ]  Winding1="[ 20e3 1e-6  0.0]"  Winding2=[ 230e3 1e-6 0.15]  Rm=500  Lm=500  L0=0.5  Saturation="[ 0,0  ;  0.005,1.2  ;  1.0,1.4 ]"  InitialFluxes=[ 0.8 , -0.8 , 0.7 ]  BreakLoop=off  DiscreteSolver=Trapezoidal iterative  DataType=off  TransfoNumber=0
  Vref1 : Constant  Value=PSSMODEL
  Vref3 : Constant
  Vref4 : Constant
  Vref5 : Constant  Value=0
  sig1 : Subsystem
  sig2 : Subsystem
  A : PMIOPort  Side=Left
  B : PMIOPort  Port=2  Side=Left
  C : PMIOPort  Port=3  Side=Left
  wires:
  Pref3/1 -> M3: Turbine & Regulators/2(Pref)
  Vref3/1 -> M3: Turbine & Regulators/3(Vref)
  Pref4/1 -> M4: Turbine & Regulators/2(Pref)
  Vref4/1 -> M4: Turbine & Regulators/3(Vref)
  Vref5/1 -> M4: Turbine & Regulators/4(PSS)
  M3 900 MVA/1 -> [m3]
  M4 900 MVA/1 -> [m4]
  sig2/1(Out1) -> M3: Turbine & Regulators/1(m)
  sig1/1(Out1) -> M4: Turbine & Regulators/1(m)
  [m4] -> sig1/1(In1)
  [m3] -> sig2/1(In1)
  Vref1/1 -> M3: Turbine & Regulators/4(PSS)
  M3: Turbine & Regulators/1(Pm) -> M3 900 MVA/1
  M3: Turbine & Regulators/2(Vf) -> M3 900 MVA/2
  M4: Turbine & Regulators/1(Pm) -> M4 900 MVA/1
  M4: Turbine & Regulators/2(Vf) -> M4 900 MVA/2
  connections:
  T3: 900MVA 20 kV-230 kV/LConn3 -- BG3/RConn3 -- Snubber/LConn3
  T3: 900MVA 20 kV-230 kV/LConn2 -- BG3/RConn2 -- Snubber/LConn2
  Snubber/LConn1 -- Load Flow Bus/LConn1 -- T3: 900MVA 20 kV-230 kV/LConn1 -- BG3/RConn1
  T3: 900MVA 20 kV-230 kV/RConn3 -- 25km Area 2/LConn3
  T4: 900MVA 20 kV/230 kV/LConn3 -- Snubber1/LConn3 -- BG4/RConn3
  T4: 900MVA 20 kV/230 kV/LConn2 -- Snubber1/LConn2 -- BG4/RConn2
  Snubber1/LConn1 -- Load Flow Bus1/LConn1 -- BG4/RConn1 -- T4: 900MVA 20 kV/230 kV/LConn1
  T3: 900MVA 20 kV-230 kV/RConn2 -- 25km Area 2/LConn2
  T3: 900MVA 20 kV-230 kV/RConn1 -- 25km Area 2/LConn1
  25km Area 2/RConn2 -- 10 km Area 2/LConn2 -- T4: 900MVA 20 kV/230 kV/RConn2
  25km Area 2/RConn1 -- 10 km Area 2/LConn1 -- T4: 900MVA 20 kV/230 kV/RConn1
  25km Area 2/RConn3 -- 10 km Area 2/LConn3 -- T4: 900MVA 20 kV/230 kV/RConn3
  M3 900 MVA/RConn1 -- BG3/LConn1
  M3 900 MVA/RConn2 -- BG3/LConn2
  M3 900 MVA/RConn3 -- BG3/LConn3
  M4 900 MVA/RConn1 -- BG4/LConn1
  M4 900 MVA/RConn2 -- BG4/LConn2
  M4 900 MVA/RConn3 -- BG4/LConn3
  10 km Area 2/RConn1 -- A/RConn1 -- -350MVAR/LConn1 -- 1767MW 100MVAR -187MVAR/LConn1
  10 km Area 2/RConn2 -- 1767MW 100MVAR -187MVAR/LConn2 -- -350MVAR/LConn2 -- B/RConn1
  10 km Area 2/RConn3 -- -350MVAR/LConn3 -- C/RConn1 -- 1767MW 100MVAR -187MVAR/LConn3

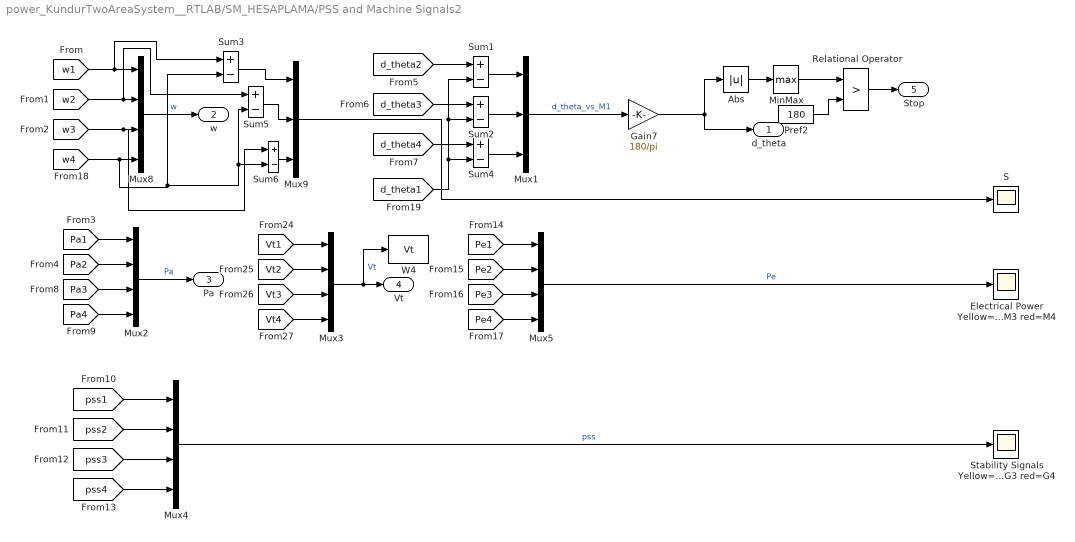
== system power_KundurTwoAreaSystem__RTLAB/SM_HESAPLAMA/PSS and Machine Signals2 ==
  Abs : Abs  SaturateOnIntegerOverflow=on
  "Electrical Power Yellow=M1 mag=M2 cyan=M3 red=M4 " : Scope
  Gain7 : Gain  Gain=180/pi
  MinMax : MinMax  Function=max  InputSameDT=on  SaturateOnIntegerOverflow=on
  Mux1 : Mux  Inputs=3
  Mux{2..5,8} (5 alike) : Mux
  Mux9 : Mux  Inputs=3
  Pref2 : Constant  Value=180
  Relational Operator : RelationalOperator  Operator=>  RndMeth=Nearest  InputSameDT=on
  S : Scope
  "Stability Signals Yellow=G1 mag=G2 cyan=G3 red=G4 " : Scope
  Sum{1..6} (6 alike) : Sum  Inputs=+-  InputSameDT=on  SaturateOnIntegerOverflow=on  OutDataTypeStr=Inherit: Same as first input
  W4 : ToWorkspace  VariableName=Vt  SampleTime=-1
  d_theta : Outport  VectorParamsAs1DForOutWhenUnconnected=off
  w : Outport  Port=2  VectorParamsAs1DForOutWhenUnconnected=off
  Pa : Outport  Port=3  VectorParamsAs1DForOutWhenUnconnected=off
  Vt : Outport  Port=4  VectorParamsAs1DForOutWhenUnconnected=off
  Stop : Outport  Port=5  VectorParamsAs1DForOutWhenUnconnected=off
  wires:
  [Pa1] -> Mux2/1
  Mux4/1 -> "Stability Signals Yellow=G1 mag=G2 cyan=G3 red=G4 "/1  "pss"
  [pss1] -> Mux4/1
  [pss2] -> Mux4/2
  [pss4] -> Mux4/4
  [pss3] -> Mux4/3
  Mux8/1 -> w/1  "w"
  Relational Operator/1 -> Stop/1
  Mux2/1 -> Pa/1  "Pa"
  [Pa2] -> Mux2/2
  [Pa3] -> Mux2/3
  [Pa4] -> Mux2/4
  [Vt1] -> Mux3/1
  [Vt2] -> Mux3/2
  [Vt3] -> Mux3/3
  [Vt4] -> Mux3/4
  Mux3/1 -> Vt/1, W4/1  "Vt"
  [Pe1] -> Mux5/1
  [Pe2] -> Mux5/2
  [Pe3] -> Mux5/3
  [Pe4] -> Mux5/4
  Mux5/1 -> "Electrical Power Yellow=M1 mag=M2 cyan=M3 red=M4 "/1  "Pe"
  [w1] -> Sum3/1, Mux8/1
  [w2] -> Sum5/1, Mux8/2
  [w3] -> Sum6/1, Mux8/3
  [w4] -> Sum3/2, Sum6/2, Sum5/2, Mux8/4
  Sum3/1 -> Mux9/1
  Sum5/1 -> Mux9/2
  Sum6/1 -> Mux9/3
  Mux9/1 -> S/1
  Mux1/1 -> Gain7/1  "d_theta_vs_M1"
  Abs/1 -> MinMax/1
  Pref2/1 -> Relational Operator/2
  MinMax/1 -> Relational Operator/1
  [d_theta2] -> Sum1/1
  Sum1/1 -> Mux1/1
  [d_theta3] -> Sum2/1
  [d_theta4] -> Sum4/1
  [d_theta1] -> Sum4/2, Sum2/2, Sum1/2
  Sum2/1 -> Mux1/2
  Sum4/1 -> Mux1/3
  Gain7/1 -> d_theta/1, Abs/1

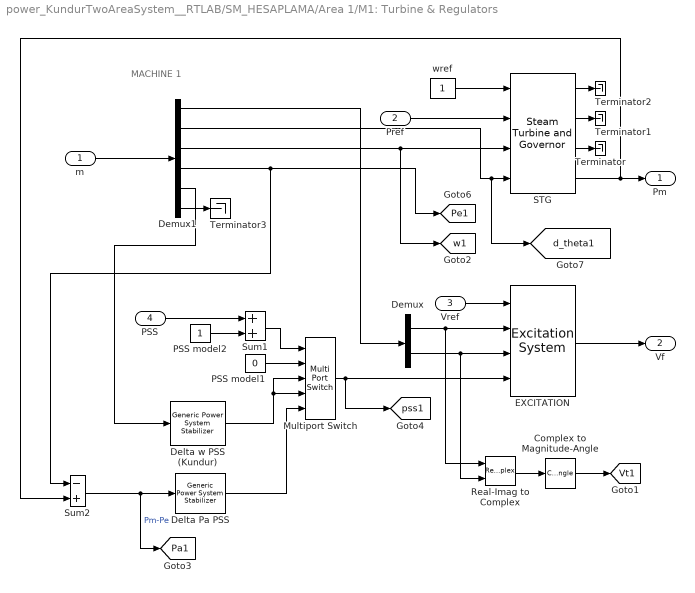
== system power_KundurTwoAreaSystem__RTLAB/SM_HESAPLAMA/Area 1/M1: Turbine & Regulators ==
  note: MACHINE 1
  m : Inport
  Pref : Inport  Port=2
  Vref : Inport  Port=3
  PSS : Inport  Port=4
  Complex to Magnitude-Angle : ComplexToMagnitudeAngle  Output=Magnitude
  Delta Pa PSS : spsGenericPowerSystemStabilizerLib/Generic Power System Stabilizer  Tsensor=15e-3  K=2.5*1.25  Twashout=1  Tleadlag1=[60e-3 1]  Tleadlag2=[0 0]  VSlimits=[-0.15 0.15]  Vinit=0  Plot_On=off  MagdB_On=on  FreqRange=logspace(-2,2,500)
      settings: SourceProductBaseCode=PS
  Delta w PSS (Kundur) : spsGenericPowerSystemStabilizerLib/Generic Power System Stabilizer  Tsensor=15e-3  K=30  Twashout=10  Tleadlag1=[50e-3 20e-3]  Tleadlag2=[3 5.4]  VSlimits=[-0.15 0.15]  Vinit=0  Plot_On=off  MagdB_On=on  FreqRange=logspace(-2,2,500)
      settings: SourceProductBaseCode=PS
  Demux : Demux  Outputs=2
      settings: DisplayOption=none
  Demux1 : Demux  Outputs=[2 1 1 1 1 1]
  EXCITATION : spsExcitationSystemLib/Excitation System  tr=20e-3  reg=[ 200, 0.001 ]  exc=[ 1, 0 ]  tgr=[ 0, 0 ]  damp=[ 0, 0 ]  sat=[ 0, 0 ]  lim=[-12.3 , 12.3, 0 ]  v0=[1,1.83395]
      settings: SourceProductBaseCode=PS
  Multiport Switch : MultiPortSwitch  Inputs=4  InputSameDT=on
  PSS model1 : Constant  Value=0
  PSS model2 : Constant
  Real-Imag to Complex : RealImagToComplex
  STG : spsSteamTurbineandGovernorLib/Steam Turbine and Governor  gentype=Tandem-compound (single mass)  reg1="[ 1  0.05    0 ]"  reg2="[ 0.001  0.15 ]"  reg3="[ -0.1  0.1  0  4.496 ]"  N=3600  turb1="[ 0  10   3.3   0.5   ]"  turb2="[   0   0.36    0.36   0.28   ]"  HA="[ 0.046  1.430  1.465   0.192 ]"  KA="[ 90.44  53.88  64.59   62.94  ]"  DA="[ 0.0115  0.3575  0.3663   0.0137  ]"  ini1=0.7778  ini2=[0.779316,-31.4247]
      settings: SourceProductBaseCode=PS
  Sum1 : Sum  InputSameDT=on  SaturateOnIntegerOverflow=on  OutDataTypeStr=Inherit: Same as first input
  Sum2 : Sum  Inputs=-+  InputSameDT=on  SaturateOnIntegerOverflow=on  OutDataTypeStr=Inherit: Same as first input
  Terminator{,1..3} (4 alike) : Terminator
  wref : Constant
  Pm : Outport  InitialOutput=0  VectorParamsAs1DForOutWhenUnconnected=off
  Vf : Outport  Port=2  InitialOutput=0  VectorParamsAs1DForOutWhenUnconnected=off
  tag scope: Pa1=global, Pe1=global, Vt1=global, d_theta1=global, pss1=global, w1=global
  wires:
  Demux/1 -> Real-Imag to Complex/1, EXCITATION/2
  Demux/2 -> Real-Imag to Complex/2, EXCITATION/3
  wref/1 -> STG/1
  Pref/1 -> STG/2
  m/1 -> Demux1/1
  Vref/1 -> EXCITATION/1
  Real-Imag to Complex/1 -> Complex to Magnitude-Angle/1
  EXCITATION/1 -> Vf/1
  Complex to Magnitude-Angle/1 -> [Vt1]
  Demux1/6 -> Terminator3/1
  PSS model1/1 -> Multiport Switch/2
  Delta w PSS (Kundur)/1 -> Multiport Switch/4, Multiport Switch/3
  Delta Pa PSS/1 -> Multiport Switch/5
  PSS model2/1 -> Sum1/2
  Sum1/1 -> Multiport Switch/1
  PSS/1 -> Sum1/1
  Demux1/1 -> Demux/1
  Demux1/3 -> [w1], STG/3
  Demux1/4 -> Sum2/1, [Pe1]
  Demux1/5 -> Delta w PSS (Kundur)/1
  Sum2/1 -> Delta Pa PSS/1, [Pa1]  "Pm-Pe"
  STG/3 -> Terminator/1
  Demux1/2 -> [d_theta1], STG/4
  STG/4 -> Pm/1, Sum2/2
  STG/2 -> Terminator1/1
  STG/1 -> Terminator2/1
  Multiport Switch/1 -> EXCITATION/4, [pss1]

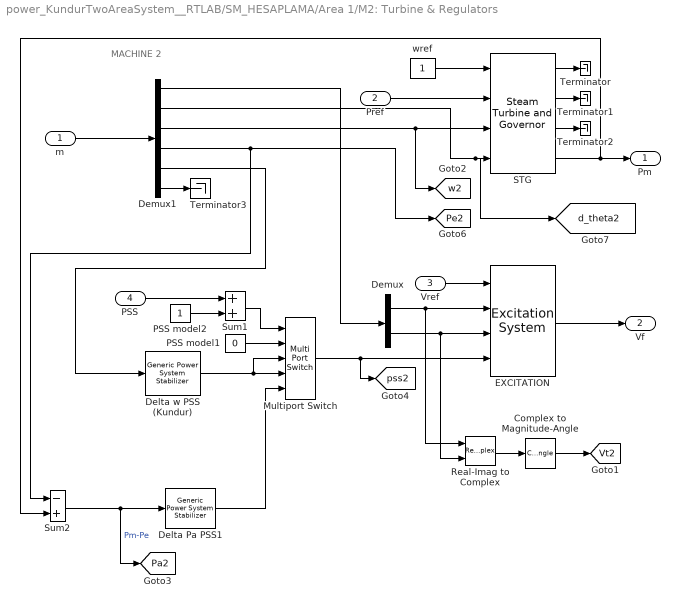
== system power_KundurTwoAreaSystem__RTLAB/SM_HESAPLAMA/Area 1/M2: Turbine & Regulators ==
  note: MACHINE 2
  m : Inport
  Pref : Inport  Port=2
  Vref : Inport  Port=3
  PSS : Inport  Port=4
  Complex to Magnitude-Angle : ComplexToMagnitudeAngle  Output=Magnitude
  Delta Pa PSS1 : spsGenericPowerSystemStabilizerLib/Generic Power System Stabilizer  Tsensor=15e-3  K=2.5*1.25  Twashout=1  Tleadlag1=[60e-3 1]  Tleadlag2=[0 0]  VSlimits=[-0.15 0.15]  Vinit=0  Plot_On=off  MagdB_On=on  FreqRange=logspace(-2,2,500)
      settings: SourceProductBaseCode=PS
  Delta w PSS (Kundur) : spsGenericPowerSystemStabilizerLib/Generic Power System Stabilizer  Tsensor=15e-3  K=30  Twashout=10  Tleadlag1=[50e-3 20e-3]  Tleadlag2=[3 5.4]  VSlimits=[-0.15 0.15]  Vinit=0  Plot_On=off  MagdB_On=on  FreqRange=logspace(-2,2,500)
      settings: SourceProductBaseCode=PS
  Demux : Demux  Outputs=2
      settings: DisplayOption=none
  Demux1 : Demux  Outputs=[2 1 1 1 1 1]
  EXCITATION : spsExcitationSystemLib/Excitation System  tr=20e-3  reg=[ 200, 0.001 ]  exc=[ 1, 0 ]  tgr=[ 0, 0 ]  damp=[ 0, 0 ]  sat=[ 0, 0 ]  lim=[ -12 , 12, 0 ]  v0=[1,1.83395]
      settings: SourceProductBaseCode=PS
  Multiport Switch : MultiPortSwitch  Inputs=4  InputSameDT=on
  PSS model1 : Constant  Value=0
  PSS model2 : Constant
  Real-Imag to Complex : RealImagToComplex
  STG : spsSteamTurbineandGovernorLib/Steam Turbine and Governor  gentype=Tandem-compound (single mass)  reg1="[ 1  0.05    0 ]"  reg2="[ 0.001  0.15 ]"  reg3="[ -0.1  0.1  0  4.496 ]"  N=3600  turb1="[ 0  10   3.3   0.5   ]"  turb2="[   0   0.36    0.36   0.28   ]"  HA="[ 0.046  1.430  1.465   0.192 ]"  KA="[ 90.44  53.88  64.59   62.94  ]"  DA="[ 0.0115  0.3575  0.3663   0.0137  ]"  ini1=0.7777  ini2=[0.779243,-42.8075]
      settings: SourceProductBaseCode=PS
  Sum1 : Sum  InputSameDT=on  SaturateOnIntegerOverflow=on  OutDataTypeStr=Inherit: Same as first input
  Sum2 : Sum  Inputs=-+  InputSameDT=on  SaturateOnIntegerOverflow=on  OutDataTypeStr=Inherit: Same as first input
  Terminator{,1..3} (4 alike) : Terminator
  wref : Constant
  Pm : Outport  InitialOutput=0  VectorParamsAs1DForOutWhenUnconnected=off
  Vf : Outport  Port=2  InitialOutput=0  VectorParamsAs1DForOutWhenUnconnected=off
  tag scope: Pa2=global, Pe2=global, Vt2=global, d_theta2=global, pss2=global, w2=global
  wires:
  Sum2/1 -> Delta Pa PSS1/1, [Pa2]  "Pm-Pe"
  Demux1/5 -> Delta w PSS (Kundur)/1
  Demux1/4 -> Sum2/1, [Pe2]
  Demux1/3 -> [w2], STG/3
  Demux1/1 -> Demux/1
  PSS/1 -> Sum1/1
  Sum1/1 -> Multiport Switch/1
  PSS model2/1 -> Sum1/2
  Delta Pa PSS1/1 -> Multiport Switch/5
  Delta w PSS (Kundur)/1 -> Multiport Switch/4, Multiport Switch/3
  PSS model1/1 -> Multiport Switch/2
  Multiport Switch/1 -> [pss2], EXCITATION/4
  Demux1/6 -> Terminator3/1
  Complex to Magnitude-Angle/1 -> [Vt2]
  EXCITATION/1 -> Vf/1
  Real-Imag to Complex/1 -> Complex to Magnitude-Angle/1
  Vref/1 -> EXCITATION/1
  Pref/1 -> STG/2
  wref/1 -> STG/1
  Demux/2 -> Real-Imag to Complex/2, EXCITATION/3
  Demux/1 -> Real-Imag to Complex/1, EXCITATION/2
  STG/1 -> Terminator/1
  STG/2 -> Terminator1/1
  STG/3 -> Terminator2/1
  STG/4 -> Pm/1, Sum2/2
  Demux1/2 -> [d_theta2], STG/4
  m/1 -> Demux1/1

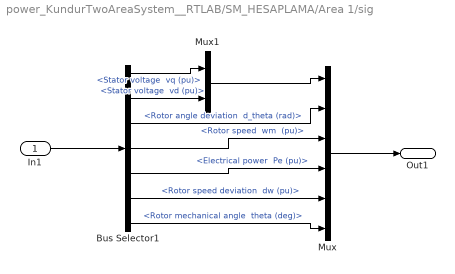
== system power_KundurTwoAreaSystem__RTLAB/SM_HESAPLAMA/Area 1/sig ==
  In1 : Inport
  Bus Selector1 : BusSelector  OutputSignals="dq0 components.Stator voltage  vq (pu),dq0 components.Stator voltage  vd (pu),Mechanical.Rotor angle deviation  d_theta (rad),Mechanical.Rotor speed  wm  (pu),Mechanical.Electrical power  Pe (pu),Mechanical.Rotor speed deviation  dw (pu),Mechanical.Rotor mechanical angle  theta (deg)"
  Mux : Mux  Inputs=6
  Mux1 : Mux  Inputs=2
  Out1 : Outport  VectorParamsAs1DForOutWhenUnconnected=off
  wires:
  Mux/1 -> Out1/1
  In1/1 -> Bus Selector1/1
  Bus Selector1/7 -> Mux/6  "<Rotor mechanical angle  theta (deg)>"
  Bus Selector1/6 -> Mux/5  "<Rotor speed deviation  dw (pu)>"
  Bus Selector1/5 -> Mux/4  "<Electrical power  Pe (pu)>"
  Bus Selector1/4 -> Mux/3  "<Rotor speed  wm  (pu)>"
  Bus Selector1/3 -> Mux/2  "<Rotor angle deviation  d_theta (rad)>"
  Bus Selector1/2 -> Mux1/2  "<Stator voltage  vd (pu)>"
  Bus Selector1/1 -> Mux1/1  "<Stator voltage  vq (pu)>"
  Mux1/1 -> Mux/1

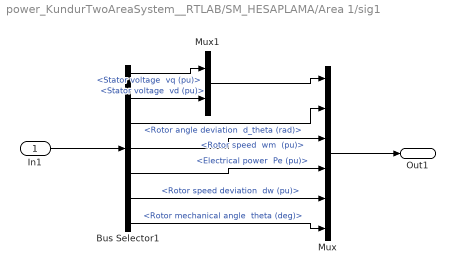
== system power_KundurTwoAreaSystem__RTLAB/SM_HESAPLAMA/Area 1/sig1 ==
  In1 : Inport
  Bus Selector1 : BusSelector  OutputSignals="dq0 components.Stator voltage  vq (pu),dq0 components.Stator voltage  vd (pu),Mechanical.Rotor angle deviation  d_theta (rad),Mechanical.Rotor speed  wm  (pu),Mechanical.Electrical power  Pe (pu),Mechanical.Rotor speed deviation  dw (pu),Mechanical.Rotor mechanical angle  theta (deg)"
  Mux : Mux  Inputs=6
  Mux1 : Mux  Inputs=2
  Out1 : Outport  VectorParamsAs1DForOutWhenUnconnected=off
  wires:
  Mux1/1 -> Mux/1
  Bus Selector1/1 -> Mux1/1  "<Stator voltage  vq (pu)>"
  Bus Selector1/2 -> Mux1/2  "<Stator voltage  vd (pu)>"
  Bus Selector1/3 -> Mux/2  "<Rotor angle deviation  d_theta (rad)>"
  Bus Selector1/4 -> Mux/3  "<Rotor speed  wm  (pu)>"
  Bus Selector1/5 -> Mux/4  "<Electrical power  Pe (pu)>"
  Bus Selector1/6 -> Mux/5  "<Rotor speed deviation  dw (pu)>"
  Bus Selector1/7 -> Mux/6  "<Rotor mechanical angle  theta (deg)>"
  In1/1 -> Bus Selector1/1
  Mux/1 -> Out1/1

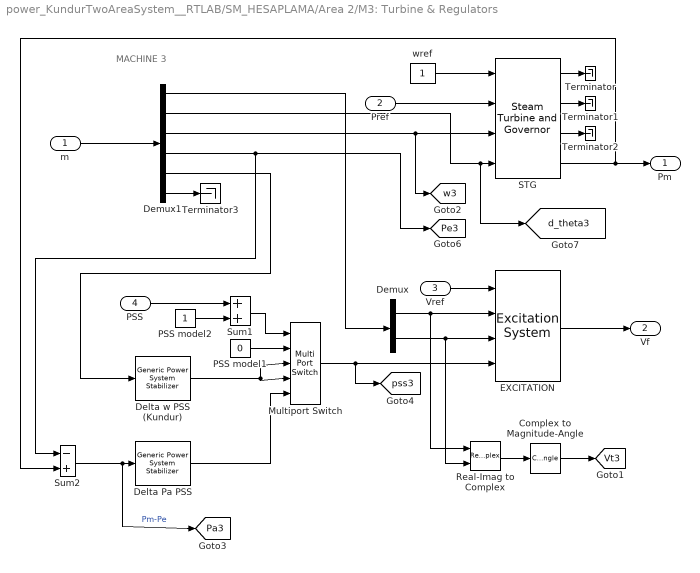
== system power_KundurTwoAreaSystem__RTLAB/SM_HESAPLAMA/Area 2/M3: Turbine & Regulators ==
  note: MACHINE 3
  m : Inport
  Pref : Inport  Port=2
  Vref : Inport  Port=3
  PSS : Inport  Port=4
  Complex to Magnitude-Angle : ComplexToMagnitudeAngle  Output=Magnitude
  Delta Pa PSS : spsGenericPowerSystemStabilizerLib/Generic Power System Stabilizer  Tsensor=15e-3  K=2.5*1.25  Twashout=1  Tleadlag1=[60e-3 1]  Tleadlag2=[0 0]  VSlimits=[-0.15 0.15]  Vinit=0  Plot_On=off  MagdB_On=on  FreqRange=logspace(-2,2,500)
      settings: SourceProductBaseCode=PS
  Delta w PSS (Kundur) : spsGenericPowerSystemStabilizerLib/Generic Power System Stabilizer  Tsensor=15e-3  K=30  Twashout=10  Tleadlag1=[50e-3 20e-3]  Tleadlag2=[3 5.4]  VSlimits=[-0.15 0.15]  Vinit=0  Plot_On=off  MagdB_On=on  FreqRange=logspace(-2,2,500)
      settings: SourceProductBaseCode=PS
  Demux : Demux  Outputs=2
      settings: DisplayOption=none
  Demux1 : Demux  Outputs=[2 1 1 1 1 1]
  EXCITATION : spsExcitationSystemLib/Excitation System  tr=20e-3  reg=[ 200, 0.001 ]  exc=[ 1, 0 ]  tgr=[ 0, 0 ]  damp=[ 0, 0 ]  sat=[ 0, 0 ]  lim=[ -12.3 , 12.3, 0 ]  v0=[1,1.83395]
      settings: SourceProductBaseCode=PS
  Multiport Switch : MultiPortSwitch  Inputs=4  InputSameDT=on
  PSS model1 : Constant  Value=0
  PSS model2 : Constant
  Real-Imag to Complex : RealImagToComplex
  STG : spsSteamTurbineandGovernorLib/Steam Turbine and Governor  gentype=Tandem-compound (single mass)  reg1="[ 1  0.05    0 ]"  reg2="[ 0.001  0.15 ]"  reg3="[ -0.1  0.1  0  4.496 ]"  N=3600  turb1="[ 0  10   3.3   0.5   ]"  turb2="[   0   0.36    0.36   0.28   ]"  HA="[ 0.046  1.430  1.465   0.192 ]"  KA="[ 90.44  53.88  64.59   62.94  ]"  DA="[ 0.0115  0.3575  0.3663   0.0137  ]"  ini1=0.798889  ini2=[0.800505,-56.3243]
      settings: SourceProductBaseCode=PS
  Sum1 : Sum  InputSameDT=on  SaturateOnIntegerOverflow=on  OutDataTypeStr=Inherit: Same as first input
  Sum2 : Sum  Inputs=-+  InputSameDT=on  SaturateOnIntegerOverflow=on  OutDataTypeStr=Inherit: Same as first input
  Terminator{,1..3} (4 alike) : Terminator
  wref : Constant
  Pm : Outport  InitialOutput=0  VectorParamsAs1DForOutWhenUnconnected=off
  Vf : Outport  Port=2  InitialOutput=0  VectorParamsAs1DForOutWhenUnconnected=off
  tag scope: Pa3=global, Pe3=global, Vt3=global, d_theta3=global, pss3=global, w3=global
  wires:
  Sum2/1 -> [Pa3], Delta Pa PSS/1  "Pm-Pe"
  Demux1/5 -> Delta w PSS (Kundur)/1
  Demux1/4 -> Sum2/1, [Pe3]
  Demux1/3 -> [w3], STG/3
  Demux1/1 -> Demux/1
  PSS/1 -> Sum1/1
  Sum1/1 -> Multiport Switch/1
  PSS model2/1 -> Sum1/2
  Delta Pa PSS/1 -> Multiport Switch/5
  Delta w PSS (Kundur)/1 -> Multiport Switch/4, Multiport Switch/3
  PSS model1/1 -> Multiport Switch/2
  Multiport Switch/1 -> [pss3], EXCITATION/4
  Demux1/6 -> Terminator3/1
  Complex to Magnitude-Angle/1 -> [Vt3]
  EXCITATION/1 -> Vf/1
  Real-Imag to Complex/1 -> Complex to Magnitude-Angle/1
  Vref/1 -> EXCITATION/1
  m/1 -> Demux1/1
  Pref/1 -> STG/2
  wref/1 -> STG/1
  Demux/2 -> Real-Imag to Complex/2, EXCITATION/3
  Demux/1 -> Real-Imag to Complex/1, EXCITATION/2
  Demux1/2 -> [d_theta3], STG/4
  STG/1 -> Terminator/1
  STG/2 -> Terminator1/1
  STG/3 -> Terminator2/1
  STG/4 -> Pm/1, Sum2/2

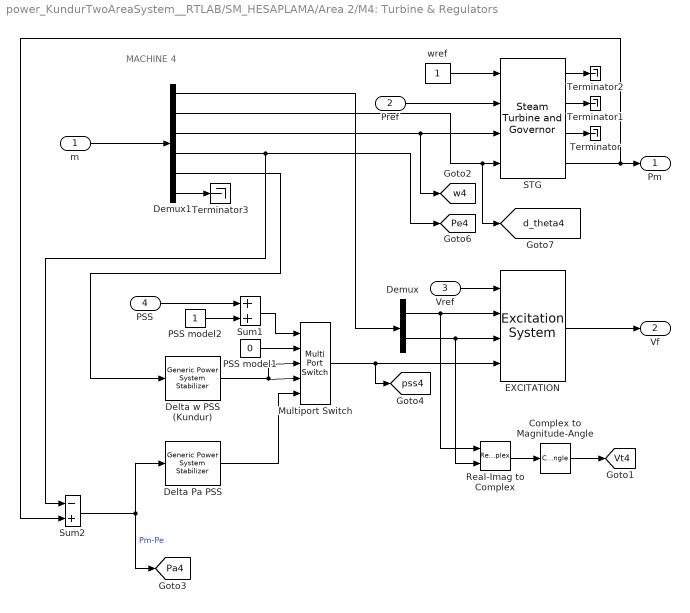
== system power_KundurTwoAreaSystem__RTLAB/SM_HESAPLAMA/Area 2/M4: Turbine & Regulators ==
  note: MACHINE 4
  m : Inport
  Pref : Inport  Port=2
  Vref : Inport  Port=3
  PSS : Inport  Port=4
  Complex to Magnitude-Angle : ComplexToMagnitudeAngle  Output=Magnitude
  "Delta Pa PSS " : spsGenericPowerSystemStabilizerLib/Generic Power System Stabilizer  Tsensor=15e-3  K=2.5*1.25  Twashout=1  Tleadlag1=[60e-3 1]  Tleadlag2=[0 0]  VSlimits=[-0.15 0.15]  Vinit=0  Plot_On=off  MagdB_On=on  FreqRange=logspace(-2,2,500)
      settings: SourceProductBaseCode=PS
  Delta w PSS (Kundur) : spsGenericPowerSystemStabilizerLib/Generic Power System Stabilizer  Tsensor=15e-3  K=30  Twashout=10  Tleadlag1=[50e-3 20e-3]  Tleadlag2=[3 5.4]  VSlimits=[-0.15 0.15]  Vinit=0  Plot_On=off  MagdB_On=on  FreqRange=logspace(-2,2,500)
      settings: SourceProductBaseCode=PS
  Demux : Demux  Outputs=2
      settings: DisplayOption=none
  Demux1 : Demux  Outputs=[2 1 1 1 1 1]
  EXCITATION : spsExcitationSystemLib/Excitation System  tr=20e-3  reg=[ 200, 0.001 ]  exc=[ 1, 0 ]  tgr=[ 0, 0 ]  damp=[ 0, 0 ]  sat=[ 0, 0 ]  lim=[ -12.3 , 12.3, 0 ]  v0=[1,1.83395]
      settings: SourceProductBaseCode=PS
  Multiport Switch : MultiPortSwitch  Inputs=4  InputSameDT=on
  PSS model1 : Constant  Value=0
  PSS model2 : Constant
  Real-Imag to Complex : RealImagToComplex
  STG : spsSteamTurbineandGovernorLib/Steam Turbine and Governor  gentype=Tandem-compound (single mass)  reg1="[ 1  0.05    0 ]"  reg2="[ 0.001  0.15 ]"  reg3="[ -0.1  0.1  0  4.496 ]"  N=3600  turb1="[ 0  10   3.3   0.5   ]"  turb2="[   0   0.36    0.36   0.28   ]"  HA="[ 0.046  1.430  1.465   0.192 ]"  KA="[ 90.44  53.88  64.59   62.94  ]"  DA="[ 0.0115  0.3575  0.3663   0.0137  ]"  ini1=0.7778  ini2=[0.779311,-67.7513]
      settings: SourceProductBaseCode=PS
  Sum1 : Sum  InputSameDT=on  SaturateOnIntegerOverflow=on  OutDataTypeStr=Inherit: Same as first input
  Sum2 : Sum  Inputs=-+  InputSameDT=on  SaturateOnIntegerOverflow=on  OutDataTypeStr=Inherit: Same as first input
  Terminator{,1..3} (4 alike) : Terminator
  wref : Constant
  Pm : Outport  InitialOutput=0  VectorParamsAs1DForOutWhenUnconnected=off
  Vf : Outport  Port=2  InitialOutput=0  VectorParamsAs1DForOutWhenUnconnected=off
  tag scope: Pa4=global, Pe4=global, Vt4=global, d_theta4=global, pss4=global, w4=global
  wires:
  Demux/1 -> Real-Imag to Complex/1, EXCITATION/2
  Demux/2 -> Real-Imag to Complex/2, EXCITATION/3
  STG/4 -> Pm/1, Sum2/2
  wref/1 -> STG/1
  Pref/1 -> STG/2
  m/1 -> Demux1/1
  Vref/1 -> EXCITATION/1
  STG/3 -> Terminator/1
  Real-Imag to Complex/1 -> Complex to Magnitude-Angle/1
  EXCITATION/1 -> Vf/1
  Complex to Magnitude-Angle/1 -> [Vt4]
  Demux1/6 -> Terminator3/1
  Multiport Switch/1 -> EXCITATION/4, [pss4]
  PSS model1/1 -> Multiport Switch/2
  Delta w PSS (Kundur)/1 -> Multiport Switch/4, Multiport Switch/3
  "Delta Pa PSS "/1 -> Multiport Switch/5
  PSS model2/1 -> Sum1/2
  Sum1/1 -> Multiport Switch/1
  PSS/1 -> Sum1/1
  Demux1/1 -> Demux/1
  Demux1/3 -> [w4], STG/3
  Demux1/4 -> Sum2/1, [Pe4]
  Demux1/5 -> Delta w PSS (Kundur)/1
  Sum2/1 -> "Delta Pa PSS "/1, [Pa4]  "Pm-Pe"
  STG/2 -> Terminator1/1
  STG/1 -> Terminator2/1
  Demux1/2 -> [d_theta4], STG/4
